simulink model "testing_new_board"  (R2024a)
settings: Solver=FixedStepAuto  StartTime=0.0  StopTime=10.0  RelTol=1e-3  EnableMultiTasking=on
libraries: stm32f4xxblockslib x1, simulink x1, stm32blockslib x1
settings Model: STM32="{\"DigitalPortWrite\":{\"ID\":\"testing_new_board:4\"},\"FDCANWrite\":{\"ID\":\"testing_new_board:1\"}}"  Creator=ezeki  LastModifiedBy=ezeki
settings SolverCC: PositivePriorityOrder=on
settings OptimizationCC: EnhancedBackFolding=on  PassReuseOutputArgsAs=Individual arguments  ZeroExternalMemoryAtStartup=off  ZeroInternalMemoryAtStartup=off  MaxStackSize=512  OptimizeBlockOrder=speed  DifferentSizesBufferReuse=on  OptimizationCustomize=off  EfficientTunableParamExpr=on
settings DebuggingCC: ParameterTunabilityLossMsg=error
settings HardwareCC: ProdBitPerPointer=32  ProdBitPerSizeT=32  ProdBitPerPtrDiffT=32  ProdLargestAtomicInteger=Long  ProdLargestAtomicFloat=Double  ProdWordSize=32  ProdLongLongMode=on  ProdHWDeviceType=ARM Compatible->ARM Cortex-M
settings SFSimCC: MATLABDynamicMemAlloc=off
settings RTWCC: Description=Embedded Coder  SystemTargetFile=ert.tlc  HardwareBoard=STM32H7xx Based (Single-core)  TLCOptions="-aInlineSetEventsForThisBaseRateFcn=TLC_FALSE -aSuppressMultiTaskScheduler=TLC_FALSE  -aRateBasedStepFcn=0"  TemplateMakefile=ert_default_tmf  Toolchain=GNU Tools for ARM Embedded Processors
settings CodeAppCC: ForceParamTrailComments=on  IgnoreCustomStorageClasses=off  OperatorAnnotations=on  SimulinkDataObjDesc=on  SFDataObjDesc=on  InsertBlockDesc=on
settings ERTTargetCC: TargetLangStandard=C99 (ISO)  CodeReplacementLibrary=ARM Cortex-M  ExtModeTransport=3  ExtModeStaticAlloc=on  ExtModeStaticAllocSize=2048  ExtModeMexFile=ext_xcp  ExtModeIntrfLevel=Level2 - Open

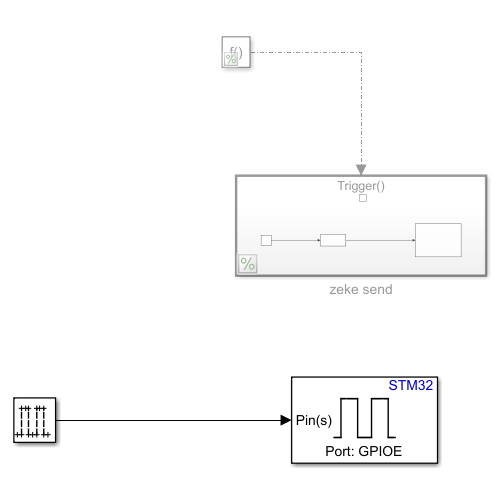
[thumbnail: Simulink's stored preview of the top-level diagram]
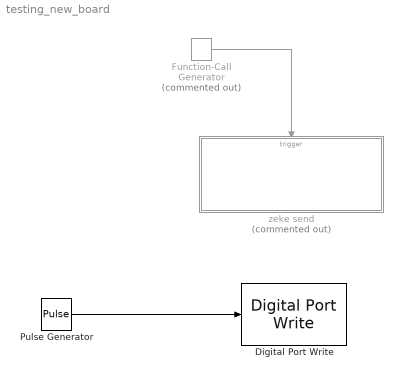
== system testing_new_board ==
  Digital Port Write : stm32f4xxblockslib/Digital Port Write  PortName=GPIOE  PinNumber=[4]  ReadOperation=off  IOAsArray=on  EnableSimPort=off  hoistedMaskSrc=ECSoC/ECSimCodegen/Digital Port Write
      settings: LibrarySourceBlock=stm32h7xxblockslib/Digital Port Write
  Function-Call Generator : simulink/Ports & Subsystems/Function-Call Generator  Commented=on  sample_time=0.1  numberOfIterations=1  DisallowWideOutput=off
  Pulse Generator : DiscretePulseGenerator  Period=4  PulseWidth=2  SampleTime=0.5
  zeke send : Subsystem  Commented=on  TreatAsAtomicUnit=on
  wires:
  Pulse Generator/1 -> Digital Port Write/1
  Function-Call Generator/1 -> zeke send/Trigger

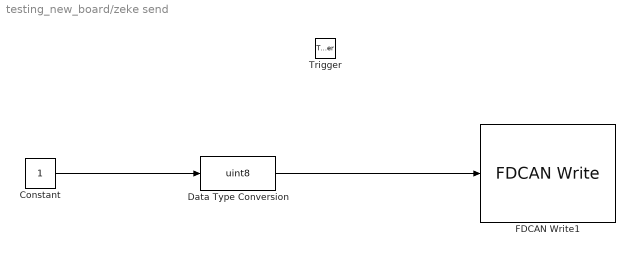
== system testing_new_board/zeke send ==
  Trigger : TriggerPort  TriggerType=function-call  VariantControl=(inherit)
  Constant : Constant
  Data Type Conversion : DataTypeConversion  OutDataTypeStr=uint8  SaturateOnIntegerOverflow=off  RndMeth=Floor
  FDCAN Write1 : stm32blockslib/FDCAN Write  FDCANModule=FDCAN1  BlockMode=Transmit  OperationReadMode=Data  OperationWriteMode=Data  ReadSource=FIFO 0  BufferNumber=0  OutputTypeReadMode=Unpacked  DataFormatWriteMode=Raw data  CANFrameType=CAN  IdentifierTypeVia=Dialog  IdentifierType=Standard (11-bit identifier)  IdentifierVia=Dialog  Identifier=529  DataLengthVia=Dialog  DataLength=1  OutputIdType=off  IsBitRateSwitchingEnabled=off  TransmitRemoteFrame=off  OutputFrameType=off  OutputBRS=off  OutputRemoteFrame=off  OutputTxFifoLevel=off  OutputRxFifoLevel=off  OutputStatus=off  Timeout=1  SampleTime=-1
      settings: LibrarySourceBlock=stm32l5xxblockslib/FDCAN Write
  wires:
  Data Type Conversion/1 -> FDCAN Write1/1
  Constant/1 -> Data Type Conversion/1
